simulink model "exampleEnergyTapping"  (Simulink 7.6)
settings: Solver=ode45  StartTime=0.0  StopTime=24*3600  MaxStep=60  RelTol=1e-3
libraries: carnot x7
settings Model: Creator=drhf  LastModifiedBy=drhf
settings CodeAppCC: CustomSymbolStrType=$N$R$M_T

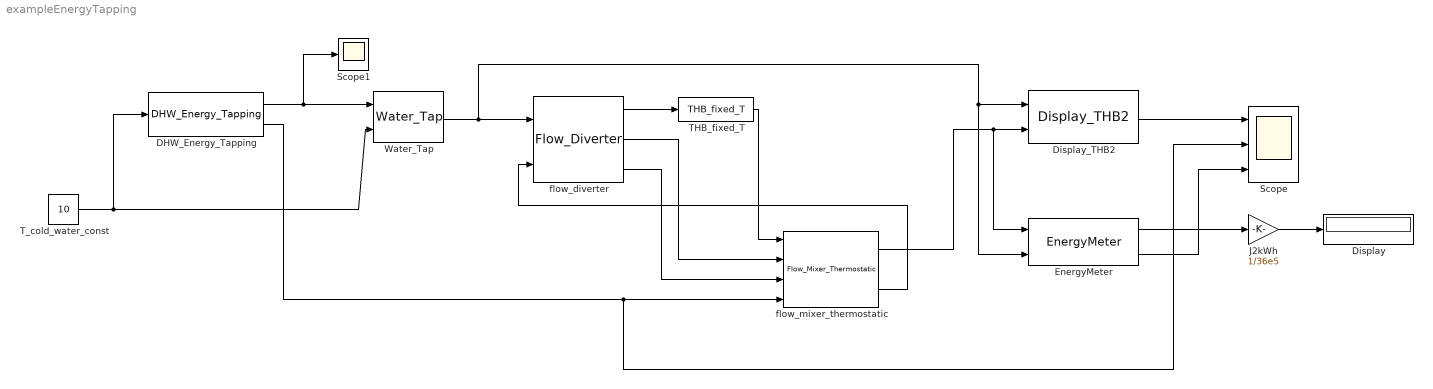
== system exampleEnergyTapping ==
  DHW_Energy_Tapping : carnot/Load/Hot_Water_Tapping/DHW_Energy_Tapping  SystemSampleTime=-1  mdot_nom=1/60  times="[7     7.1 7.5   8.083 8.25  8.5   8.75  9     9.5   10.5  11.5  11.75 12.75 14.5  15.5  16.5  18    18.25 18.5  19    20.5  21.25 21.5]*3600"  energies=[0.105 1.4 0.105 0.105 0.105 0.105 0.105 0.105 0.105 0.105 0.105 0.105 0.315 0.105 0.105 0.105 0.105 0.105 0.105 0.105 0.735 0.105 1.4 ]*36e5  dT_set="[30    30  30    30    30    30    30    30    30    30    30    30    45    30    30    30    30    30    30    30    45    30    30  ]"  coeffs="[3     6   3     3     3     3     3     3     3     3     3     3     4     3     3     3     3     3     3     3     4     3     6   ]"
  Display : Display
  Display_THB2 : carnot/Outputs/Display_THB2  SystemSampleTime=-1  t=off  m=on  p=off  id=off  mix=off  d=off
  EnergyMeter : carnot/Control/EnergyMeter  SystemSampleTime=-1
  J2kWh : Gain  Gain=1/36e5
  Scope : Scope  NumInputPorts=3
      settings: YMin=-5~-5~-5  YMax=5~5~5
  Scope1 : Scope
  THB_fixed_T : carnot/Source/Simple/THB_fixed_T  SystemSampleTime=-1  t=60
  T_cold_water_const : Constant  Value=10
  Water_Tap : carnot/Load/Hot_Water_Tapping/Water_Tap  SystemSampleTime=-1  dia=0.02  p=2e5
  flow_diverter : carnot/Hydraulics/Flow_Diverter  SystemSampleTime=-1
  flow_mixer_thermostatic : carnot/Hydraulics/Flow_Mixer_Thermostatic  SystemSampleTime=-1  t=10
  wires:
  Display_THB2/1 -> Scope/1
  EnergyMeter/1 -> J2kWh/1
  J2kWh/1 -> Display/1
  EnergyMeter/2 -> Scope/3
  DHW_Energy_Tapping/2 -> flow_mixer_thermostatic/4, Scope/2
  flow_diverter/3 -> flow_mixer_thermostatic/3
  flow_diverter/2 -> flow_mixer_thermostatic/2
  THB_fixed_T/1 -> flow_mixer_thermostatic/1
  flow_mixer_thermostatic/1 -> Display_THB2/2, EnergyMeter/1
  flow_mixer_thermostatic/2 -> flow_diverter/2
  Water_Tap/1 -> flow_diverter/1, Display_THB2/1, EnergyMeter/2
  T_cold_water_const/1 -> Water_Tap/2, DHW_Energy_Tapping/1
  DHW_Energy_Tapping/1 -> Water_Tap/1, Scope1/1
  flow_diverter/1 -> THB_fixed_T/1
